simulink model "nxtway_gs_controller"  (Simulink 7.0)
settings: Solver=FixedStepDiscrete  SolverMode=SingleTasking  StartTime=0  StopTime=inf  FixedStep=TS  RelTol=1e-3
PreLoadFcn:
  | param_nxtway_gs
values from neighbouring files (symbols this model uses):
  a_b = 0.8    [param_controller.m]
  a_d = 0.8    [param_controller.m]
  a_gc = 0.8    [param_controller.m]
  a_gd = 0.999    [param_controller.m]
  a_r = 0.996    [param_controller.m]
  dst_thr = 20    [param_controller.m]
  gp_max = 100    [param_controller.m]
  k_f = KK(1, 1:4)    [param_controller.m]
  k_i = KK(1, 5)    [param_controller.m]
  k_phidot = 25    [param_controller.m]
  k_sync = 0.35    [param_controller.m]
  k_thetadot = 0.3 / R    [param_controller.m]
  log_count = 25    [param_controller.m]
  pwm_gain = 1    [param_controller.m]
  sound_dur = 500    [param_controller.m]
  sound_freq = 440    [param_controller.m]
  time_auto = 5000    [param_controller.m]
  time_start = 1000    [param_controller.m]
  ts1 = 0.004    [param_controller.m]
  ts2 = 0.02    [param_controller.m]
  ts3 = 0.1    [param_controller.m]
  turn_angle = round(60 * W / R)    [param_controller.m]
undefined symbols (not defined in the file or in its folder): LEJOS, OSEK
libraries: ecrobot_nxt_lib x30, simulink x2
(part 2 of 2)

== system nxtway_gs_controller/nxtway_app/task_ts1/Balance & Drive Control/Controller/Cal PWM/Cal theta_diff/Detect Flag Falling ==
  flag : Inport  OutDataType=sfix(16)  OutScaling=2^0
  Constant : Constant  Value=0  VectorParams1D=off  OutDataTypeMode=boolean  OutDataType=FIXDT  OutScaling=2^0  SampleTime=-1
      settings: AttributesFormatString=DataType = %<OutDataTypeStr>
  Constant1 : Constant  VectorParams1D=off  OutDataTypeMode=boolean  OutDataType=FIXDT  OutScaling=2^0  SampleTime=-1
      settings: AttributesFormatString=DataType = %<OutDataTypeStr>
  Logical Operator : Logic  AllPortsSameDT=off  OutDataTypeMode=boolean
  Relational Operator : RelationalOperator  Operator===  LogicOutDataTypeMode=boolean
  Relational Operator1 : RelationalOperator  Operator===  LogicOutDataTypeMode=boolean
  Unit Delay : UnitDelay  SampleTime=-1
  falling : Outport  OutDataType=sfix(16)  OutScaling=2^0
  wires:
  flag/1 -> Unit Delay/1, Relational Operator/1
  Constant/1 -> Relational Operator/2
  Unit Delay/1 -> Relational Operator1/1
  Constant1/1 -> Relational Operator1/2
  Relational Operator/1 -> Logical Operator/1
  Relational Operator1/1 -> Logical Operator/2
  Logical Operator/1 -> falling/1

== system nxtway_gs_controller/nxtway_app/task_ts1/Balance & Drive Control/Controller/Cal PWM/Cal theta_diff/Set theta_offset ==
  theta_diff : Inport
  Enable : EnablePort
  theta_offset : Outport
  wires:
  theta_diff/1 -> theta_offset/1
